simulink model "Day3_avoidance"  (R2022b)
settings: Solver=FixedStepAuto  StartTime=0.0  StopTime=inf  FixedStep=0.001  RelTol=1e-3  EnableMultiTasking=on
undefined symbols (not defined in the file): DiscIntNeverNeededParam
libraries: raspberrypiBasiclib x15, simulink x4, raspberrypisensorlib x1
settings Model: PacingRate=10  Creator=user  LastModifiedBy=user
settings SolverCC: PositivePriorityOrder=on
settings OptimizationCC: EnhancedBackFolding=on  PassReuseOutputArgsAs=Individual arguments  ZeroExternalMemoryAtStartup=off  ZeroInternalMemoryAtStartup=off  MaxStackSize=64  OptimizeBlockOrder=speed  DifferentSizesBufferReuse=on  OptimizationCustomize=off  EfficientTunableParamExpr=on
settings DebuggingCC: ParameterTunabilityLossMsg=error
settings HardwareCC: ProdBitPerPointer=32  ProdBitPerSizeT=32  ProdBitPerPtrDiffT=32  ProdLargestAtomicInteger=Long  ProdLargestAtomicFloat=Double  ProdWordSize=32  ProdLongLongMode=on  ProdHWDeviceType=ARM Compatible->ARM Cortex
settings RTWCC: Description=Embedded Coder  SystemTargetFile=ert.tlc  HardwareBoard=Raspberry Pi  TLCOptions="-aInlineSetEventsForThisBaseRateFcn=TLC_FALSE -aSuppressMultiTaskScheduler=TLC_FALSE  -aRateBasedStepFcn=0"  TemplateMakefile=ert_default_tmf  Toolchain=GNU GCC Embedded Linux  BuildConfiguration=Faster Runs
settings CodeAppCC: ForceParamTrailComments=on  IgnoreCustomStorageClasses=off  OperatorAnnotations=on  SimulinkDataObjDesc=on  SFDataObjDesc=on  InsertBlockDesc=on
settings ERTTargetCC: SupportVariableSizeSignals=on  ExtModeTransport=2  ExtModeStaticAlloc=on  ExtModeMexFile=ext_xcp  ExtModeIntrfLevel=Level2 - Open

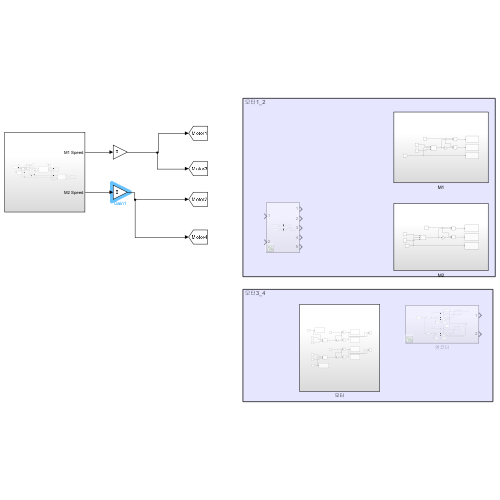
[thumbnail: Simulink's stored preview of the top-level diagram]
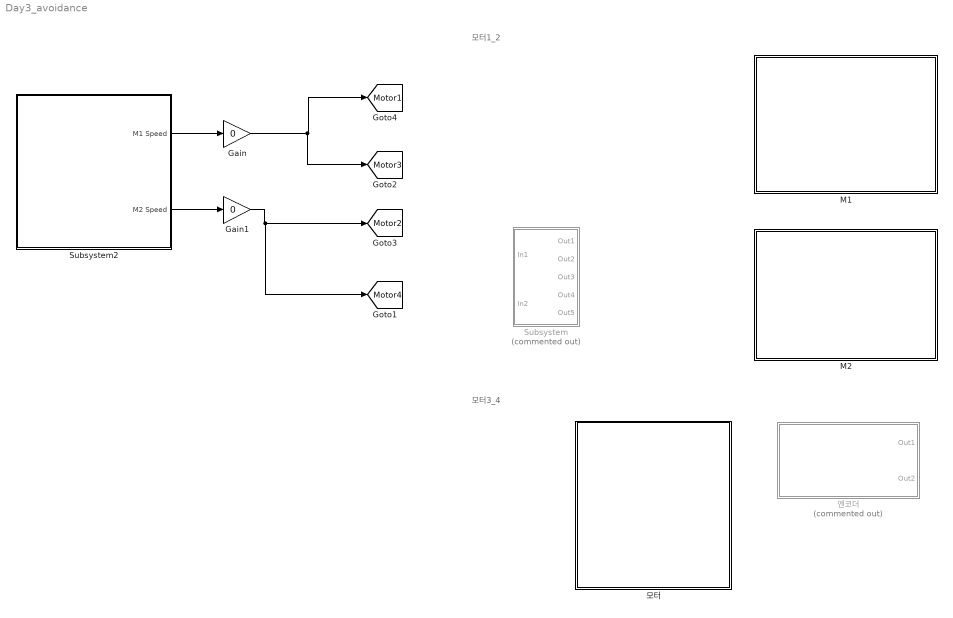
== system Day3_avoidance ==
  note: 모터1_2
  note: 모터3_4
  Gain : Gain  Gain=0
  Gain1 : Gain  Gain=0
  M1 : Subsystem
  M2 : Subsystem
  Subsystem : Subsystem  Commented=on
  Subsystem2 : Subsystem
  모터 : Subsystem
  엔코더 : Subsystem  Commented=on
  tag scope: Motor1=global, Motor2=global, Motor3=global, Motor4=global
  wires:
  Subsystem2/1(M1 Speed) -> Gain/1
  Subsystem2/2(M2 Speed) -> Gain1/1
  Gain/1 -> [Motor3], [Motor1]
  Gain1/1 -> [Motor4], [Motor2]

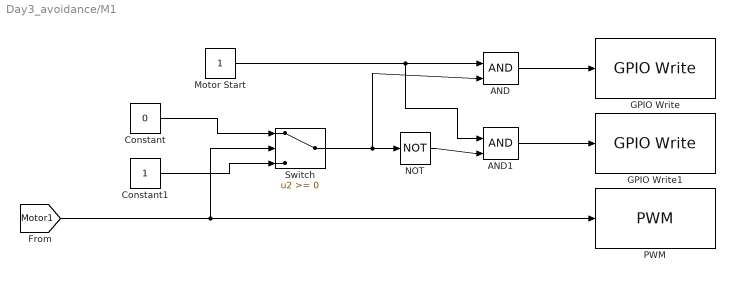
== system Day3_avoidance/M1 ==
  AND : Logic  IconShape=distinctive  AllPortsSameDT=off  OutDataTypeStr=boolean
  AND1 : Logic  IconShape=distinctive  AllPortsSameDT=off  OutDataTypeStr=boolean
  Constant : Constant  Value=0
  Constant1 : Constant
  GPIO Write : raspberrypiBasiclib/GPIO Write  board=Pi 4 Model B  gpio=15  direction=Output  blockPlatform=Raspberry Pi
  GPIO Write1 : raspberrypiBasiclib/GPIO Write  board=Pi 4 Model B  gpio=14  direction=Output  blockPlatform=Raspberry Pi
  Motor Start : Constant
  NOT : Logic  Operator=NOT  IconShape=distinctive  AllPortsSameDT=off  OutDataTypeStr=boolean
  PWM : raspberrypiBasiclib/PWM  board=Pi 4 Model B  Pin_=18  Frequency=50  blockPlatform=Raspberry Pi
  Switch : Switch  SaturateOnIntegerOverflow=off  InputSameDT=off
  wires:
  AND/1 -> GPIO Write/1
  Switch/1 -> AND/2, NOT/1
  Motor Start/1 -> AND1/1, AND/1
  AND1/1 -> GPIO Write1/1
  NOT/1 -> AND1/2
  [Motor1] -> Switch/2, PWM/1
  Constant/1 -> Switch/1
  Constant1/1 -> Switch/3

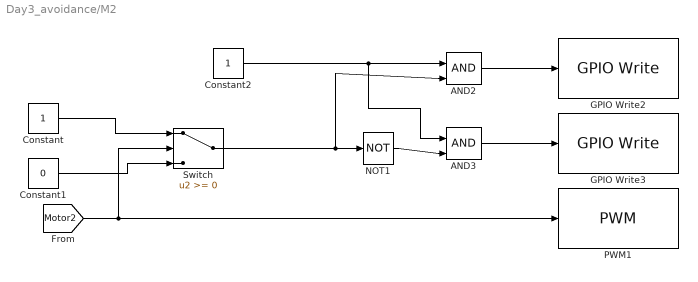
== system Day3_avoidance/M2 ==
  AND2 : Logic  IconShape=distinctive  AllPortsSameDT=off  OutDataTypeStr=boolean
  AND3 : Logic  IconShape=distinctive  AllPortsSameDT=off  OutDataTypeStr=boolean
  Constant : Constant
  Constant1 : Constant  Value=0
  Constant2 : Constant
  GPIO Write2 : raspberrypiBasiclib/GPIO Write  board=Pi 4 Model B  gpio=13  direction=Output  blockPlatform=Raspberry Pi
  GPIO Write3 : raspberrypiBasiclib/GPIO Write  board=Pi 4 Model B  gpio=6  direction=Output  blockPlatform=Raspberry Pi
  NOT1 : Logic  Operator=NOT  IconShape=distinctive  AllPortsSameDT=off  OutDataTypeStr=boolean
  PWM1 : raspberrypiBasiclib/PWM  board=Pi 4 Model B  Pin_=9  Frequency=50  blockPlatform=Raspberry Pi
  Switch : Switch  SaturateOnIntegerOverflow=off  InputSameDT=off
  wires:
  Constant2/1 -> AND3/1, AND2/1
  AND2/1 -> GPIO Write2/1
  AND3/1 -> GPIO Write3/1
  NOT1/1 -> AND3/2
  Switch/1 -> AND2/2, NOT1/1
  Constant1/1 -> Switch/3
  Constant/1 -> Switch/1
  [Motor2] -> Switch/2, PWM1/1

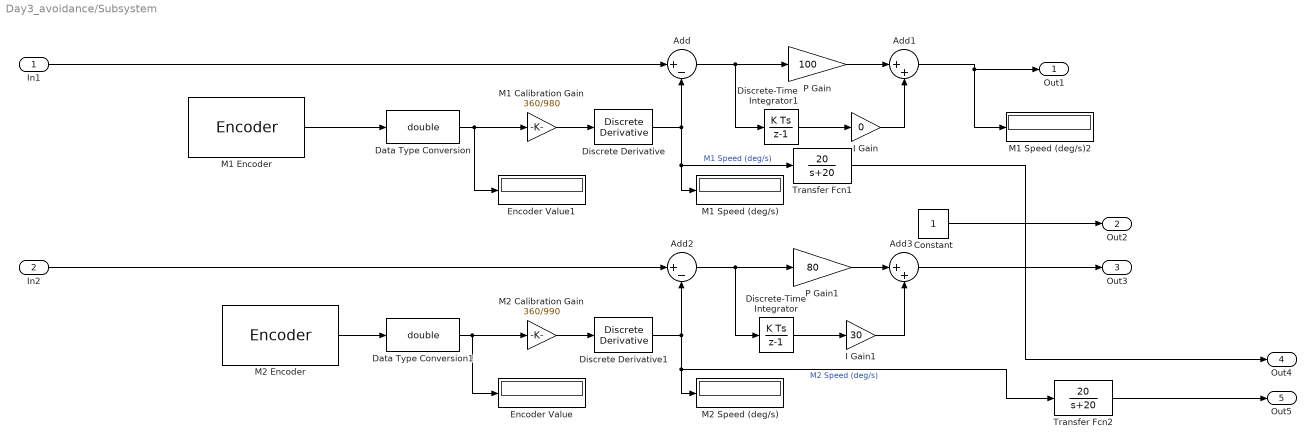
== system Day3_avoidance/Subsystem ==
  In1 : Inport
  In2 : Inport  Port=2
  Add : Sum  Inputs=|+-
  Add1 : Sum  Inputs=|++
  Add2 : Sum  Inputs=|+-
  Add3 : Sum  Inputs=|++
  Constant : Constant
  Data Type Conversion : DataTypeConversion  OutDataTypeStr=double  SaturateOnIntegerOverflow=off  RndMeth=Floor
  Data Type Conversion1 : DataTypeConversion  OutDataTypeStr=double  SaturateOnIntegerOverflow=off  RndMeth=Floor
  Discrete Derivative : simulink/Discrete/Discrete Derivative  gainval=1  ICPrevScaledInput=0.0  OutMin=[]  OutMax=[]  OutDataType=fixdt(1, 16)  OutScaling=2^-10  DoSatur=off
  Discrete Derivative1 : simulink/Discrete/Discrete Derivative  gainval=1.0  ICPrevScaledInput=0.0  OutMin=[]  OutMax=[]  OutDataType=fixdt(1, 16)  OutScaling=2^-10  DoSatur=off
  Discrete-Time Integrator : DiscreteIntegrator  SampleTime=-1  ICPrevOutput=DiscIntNeverNeededParam  ICPrevScaledInput=DiscIntNeverNeededParam
  Discrete-Time Integrator1 : DiscreteIntegrator  SampleTime=-1  ICPrevOutput=DiscIntNeverNeededParam  ICPrevScaledInput=DiscIntNeverNeededParam
  Encoder Value : Display
  Encoder Value1 : Display
  I Gain : Gain  Gain=0
  I Gain1 : Gain  Gain=30
  M1 Calibration Gain : Gain  Gain=360/980
  M1 Encoder : raspberrypiBasiclib/Encoder  BoardProperty=Pi 2 Model B  InputA=GPIO 10  InputB=GPIO 20  Mode=No reset  SampleTime=-1
  M1 Speed (deg/s) : Display
  M1 Speed (deg/s)2 : Display
  M2 Calibration Gain : Gain  Gain=360/990
  M2 Encoder : raspberrypiBasiclib/Encoder  BoardProperty=Pi 2 Model B  InputA=GPIO 17  InputB=GPIO 27  Mode=No reset  SampleTime=-1
  M2 Speed (deg/s) : Display
  P Gain : Gain  Gain=100
  P Gain1 : Gain  Gain=80
  Transfer Fcn1 : TransferFcn  Numerator=[20]  Denominator=[1 20]
  Transfer Fcn2 : TransferFcn  Numerator=[20]  Denominator=[1 20]
  Out1 : Outport
  Out2 : Outport  Port=2
  Out3 : Outport  Port=3
  Out4 : Outport  Port=4
  Out5 : Outport  Port=5
  wires:
  Discrete Derivative1/1 -> Add2/2, Transfer Fcn2/1, M2 Speed (deg/s)/1  "M2 Speed (deg/s)"
  M2 Calibration Gain/1 -> Discrete Derivative1/1
  Add1/1 -> Out1/1, M1 Speed (deg/s)2/1
  P Gain1/1 -> Add3/1
  Discrete-Time Integrator/1 -> I Gain1/1
  Add3/1 -> Out3/1
  M1 Encoder/1 -> Data Type Conversion/1
  Transfer Fcn1/1 -> Out4/1
  Transfer Fcn2/1 -> Out5/1
  In2/1 -> Add2/1
  Data Type Conversion/1 -> M1 Calibration Gain/1, Encoder Value1/1
  Constant/1 -> Out2/1
  Discrete Derivative/1 -> Add/2, Transfer Fcn1/1, M1 Speed (deg/s)/1  "M1 Speed (deg/s)"
  Discrete-Time Integrator1/1 -> I Gain/1
  Add/1 -> Discrete-Time Integrator1/1, P Gain/1
  M1 Calibration Gain/1 -> Discrete Derivative/1
  Add2/1 -> Discrete-Time Integrator/1, P Gain1/1
  I Gain1/1 -> Add3/2
  Data Type Conversion1/1 -> Encoder Value/1, M2 Calibration Gain/1
  I Gain/1 -> Add1/2
  M2 Encoder/1 -> Data Type Conversion1/1
  In1/1 -> Add/1
  P Gain/1 -> Add1/1

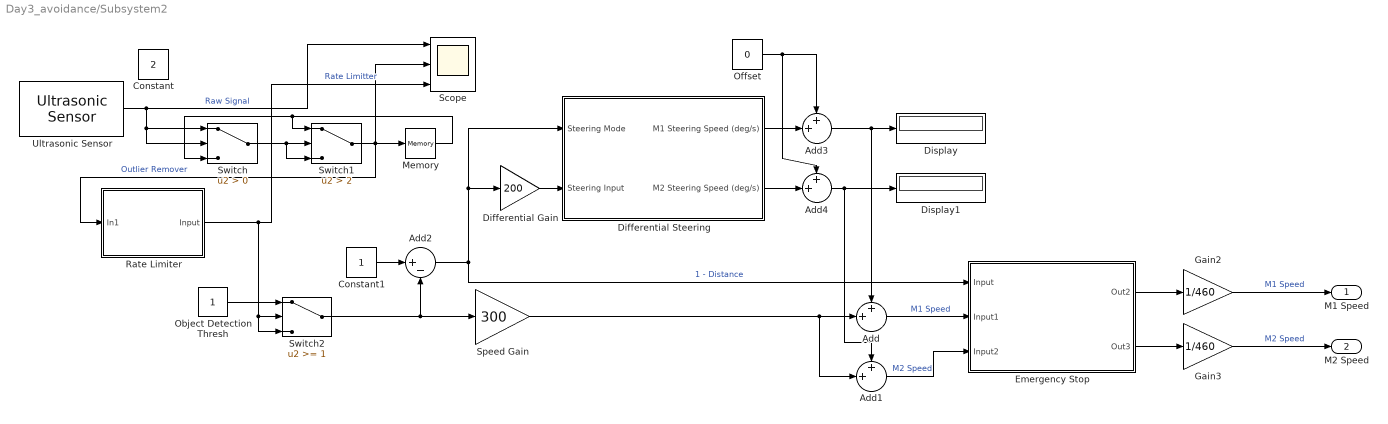
== system Day3_avoidance/Subsystem2 ==
  Add{,1,3..4} (4 alike) : Sum  Inputs=++|
  Add2 : Sum  Inputs=|+-
  Constant : Constant  Value=2
  Constant1 : Constant
  Differential Gain : Gain  Gain=200
  Differential Steering : Subsystem
  Display : Display
  Display1 : Display
  Emergency Stop : Subsystem
  Gain2 : Gain  Gain=1/460
  Gain3 : Gain  Gain=1/460
  Memory : Memory  InheritSampleTime=on  LinearizeMemory=on  LinearizeAsDelay=on
  Object Detection Thresh : Constant
  Offset : Constant  Value=0
  Rate Limiter : Subsystem
  Scope : Scope  NumInputPorts=3
  Speed Gain : Gain  Gain=300
  Switch : Switch  Criteria=u2 > Threshold  SaturateOnIntegerOverflow=off  InputSameDT=off
  Switch1 : Switch  Criteria=u2 > Threshold  Threshold=2  SaturateOnIntegerOverflow=off  InputSameDT=off
  Switch2 : Switch  Threshold=1  SaturateOnIntegerOverflow=off  InputSameDT=off
  Ultrasonic Sensor : raspberrypisensorlib/Ultrasonic Sensor  BoardProperty=Pi 4 Model B  NumSignalPins=2  TrigPin=GPIO 23  EchoPin=GPIO 24  SignalPin=GPIO 23  SampleTime=0.1  BlockPlatform=RASPBERRYPI
  M1 Speed : Outport
  M2 Speed : Outport  Port=2
  wires:
  Add3/1 -> Add/1, Display/1
  Add4/1 -> Display1/1, Add1/1
  Ultrasonic Sensor/1 -> Switch/2, Switch/1, Scope/1  "Raw Signal"
  Add2/1 -> Differential Gain/1, Differential Steering/1(Steering Mode), Emergency Stop/1(Input)  "1 - Distance"
  Differential Steering/2(M2 Steering Speed (deg/s)) -> Add4/2
  Switch/1 -> Switch1/3, Switch1/2
  Switch1/1 -> Memory/1, Scope/2, Rate Limiter/1(In1)  "Outlier Remover"
  Object Detection Thresh/1 -> Switch2/1
  Differential Steering/1(M1 Steering Speed (deg/s)) -> Add3/2
  Offset/1 -> Add4/1, Add3/1
  Gain2/1 -> M1 Speed/1  "M1 Speed"
  Constant1/1 -> Add2/1
  Differential Gain/1 -> Differential Steering/2(Steering Input)
  Gain3/1 -> M2 Speed/1  "M2 Speed"
  Switch2/1 -> Speed Gain/1, Add2/2
  Rate Limiter/1(Input) -> Scope/3, Switch2/3, Switch2/2  "Rate Limitter"
  Emergency Stop/1(Out2) -> Gain2/1
  Emergency Stop/2(Out3) -> Gain3/1
  Add/1 -> Emergency Stop/2(Input1)  "M1 Speed"
  Add1/1 -> Emergency Stop/3(Input2)  "M2 Speed"
  Memory/1 -> Switch/3, Switch1/1
  Speed Gain/1 -> Add1/2, Add/2

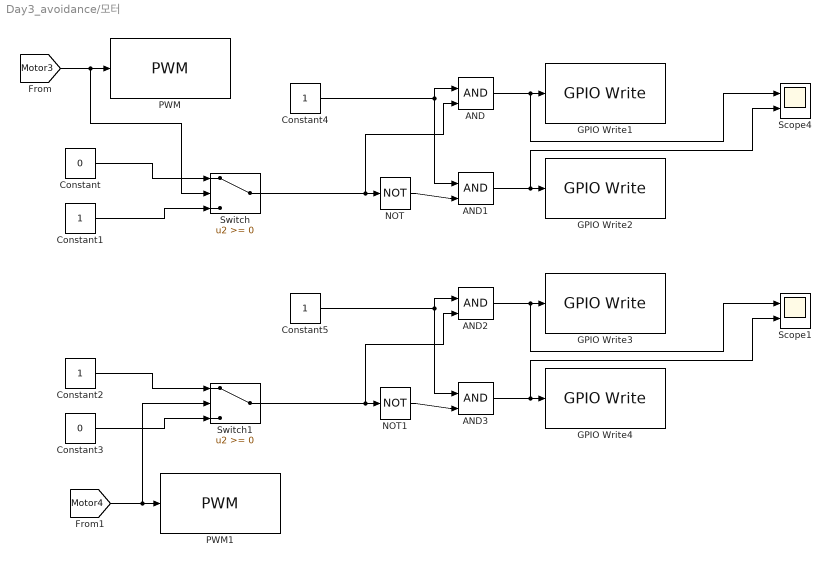
== system Day3_avoidance/모터 ==
  AND{,1..3} (4 alike) : Logic  IconShape=distinctive  AllPortsSameDT=off  OutDataTypeStr=boolean
  Constant : Constant  Value=0
  Constant{1..2,4..5} (4 alike) : Constant
  Constant3 : Constant  Value=0
  GPIO Write1 : raspberrypiBasiclib/GPIO Write  board=Pi 4 Model B  gpio=17  direction=Output  blockPlatform=Raspberry Pi
  GPIO Write2 : raspberrypiBasiclib/GPIO Write  board=Pi 4 Model B  gpio=27  direction=Output  blockPlatform=Raspberry Pi
  GPIO Write3 : raspberrypiBasiclib/GPIO Write  board=Pi 4 Model B  gpio=19  direction=Output  blockPlatform=Raspberry Pi
  GPIO Write4 : raspberrypiBasiclib/GPIO Write  board=Pi 4 Model B  gpio=26  direction=Output  blockPlatform=Raspberry Pi
  NOT : Logic  Operator=NOT  IconShape=distinctive  AllPortsSameDT=off  OutDataTypeStr=boolean
  NOT1 : Logic  Operator=NOT  IconShape=distinctive  AllPortsSameDT=off  OutDataTypeStr=boolean
  PWM : raspberrypiBasiclib/PWM  board=Pi 4 Model B  Pin_=25  Frequency=500  blockPlatform=Raspberry Pi
  PWM1 : raspberrypiBasiclib/PWM  board=Pi 4 Model B  Pin_=22  Frequency=500  blockPlatform=Raspberry Pi
  Scope1 : Scope  NumInputPorts=2
  Scope4 : Scope  NumInputPorts=2
  Switch : Switch  SaturateOnIntegerOverflow=off  InputSameDT=off
  Switch1 : Switch  SaturateOnIntegerOverflow=off  InputSameDT=off
  wires:
  Switch/1 -> AND/2, NOT/1
  Constant4/1 -> AND/1, AND1/1
  NOT/1 -> AND1/2
  AND/1 -> Scope4/1, GPIO Write1/1
  AND1/1 -> Scope4/2, GPIO Write2/1
  AND3/1 -> Scope1/2, GPIO Write4/1
  NOT1/1 -> AND3/2
  AND2/1 -> Scope1/1, GPIO Write3/1
  Constant5/1 -> AND2/1, AND3/1
  Switch1/1 -> AND2/2, NOT1/1
  [Motor3] -> Switch/2, PWM/1
  [Motor4] -> Switch1/2, PWM1/1
  Constant1/1 -> Switch/3
  Constant/1 -> Switch/1
  Constant2/1 -> Switch1/1
  Constant3/1 -> Switch1/3

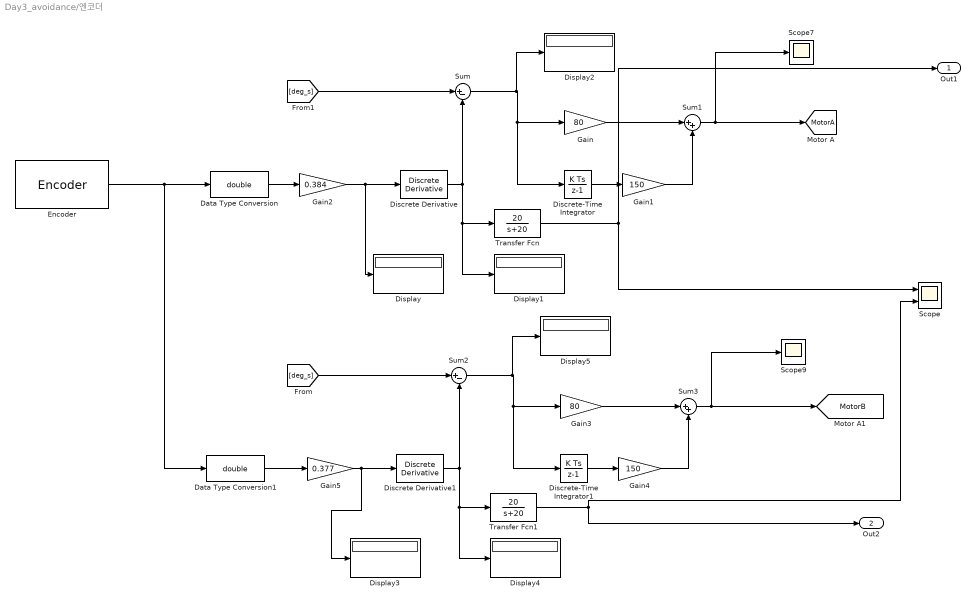
== system Day3_avoidance/엔코더 ==
  Data Type Conversion : DataTypeConversion  OutDataTypeStr=double  SaturateOnIntegerOverflow=off  RndMeth=Floor
  Data Type Conversion1 : DataTypeConversion  OutDataTypeStr=double  SaturateOnIntegerOverflow=off  RndMeth=Floor
  Discrete Derivative : simulink/Discrete/Discrete Derivative  gainval=1.0  ICPrevScaledInput=0.0  OutMin=[]  OutMax=[]  OutDataType=fixdt(1, 16)  OutScaling=2^-10  DoSatur=off
  Discrete Derivative1 : simulink/Discrete/Discrete Derivative  gainval=1.0  ICPrevScaledInput=0.0  OutMin=[]  OutMax=[]  OutDataType=fixdt(1, 16)  OutScaling=2^-10  DoSatur=off
  Discrete-Time Integrator : DiscreteIntegrator  SampleTime=-1  ICPrevOutput=DiscIntNeverNeededParam  ICPrevScaledInput=DiscIntNeverNeededParam
  Discrete-Time Integrator1 : DiscreteIntegrator  SampleTime=-1  ICPrevOutput=DiscIntNeverNeededParam  ICPrevScaledInput=DiscIntNeverNeededParam
  Display{,1..5} (6 alike) : Display
  Encoder : raspberrypiBasiclib/Encoder  BoardProperty=Pi 2 Model B  InputA=GPIO 11  InputB=GPIO 12  Mode=No reset  SampleTime=-1
  Gain : Gain  Gain=80
  Gain1 : Gain  Gain=150
  Gain2 : Gain  Gain=0.384
  Gain3 : Gain  Gain=80
  Gain4 : Gain  Gain=150
  Gain5 : Gain  Gain=0.377
  Scope : Scope  NumInputPorts=2
  Scope7 : Scope
  Scope9 : Scope
  Sum : Sum  Inputs=|+-
  Sum1 : Sum  Inputs=|++
  Sum2 : Sum  Inputs=|+-
  Sum3 : Sum  Inputs=|++
  Transfer Fcn : TransferFcn  Numerator=[20]  Denominator=[1 20]
  Transfer Fcn1 : TransferFcn  Numerator=[20]  Denominator=[1 20]
  Out1 : Outport
  Out2 : Outport  Port=2
  tag scope: MotorA=global, MotorB=global
  wires:
  Sum2/1 -> Display5/1, Discrete-Time Integrator1/1, Gain3/1
  Discrete Derivative/1 -> Transfer Fcn/1, Display1/1, Sum/2
  Discrete-Time Integrator/1 -> Gain1/1
  Gain1/1 -> Sum1/2
  Gain2/1 -> Discrete Derivative/1, Display/1
  Gain/1 -> Sum1/1
  Data Type Conversion/1 -> Gain2/1
  Sum/1 -> Display2/1, Discrete-Time Integrator/1, Gain/1
  Encoder/1 -> Data Type Conversion1/1, Data Type Conversion/1
  Sum1/1 -> [MotorA], Scope7/1
  [deg_s] -> Sum/1
  Sum3/1 -> [MotorB], Scope9/1
  Gain3/1 -> Sum3/1
  Gain4/1 -> Sum3/2
  Gain5/1 -> Discrete Derivative1/1, Display3/1
  Discrete Derivative1/1 -> Transfer Fcn1/1, Display4/1, Sum2/2
  [deg_s] -> Sum2/1
  Discrete-Time Integrator1/1 -> Gain4/1
  Data Type Conversion1/1 -> Gain5/1
  Transfer Fcn/1 -> Out1/1, Scope/1
  Transfer Fcn1/1 -> Out2/1, Scope/2

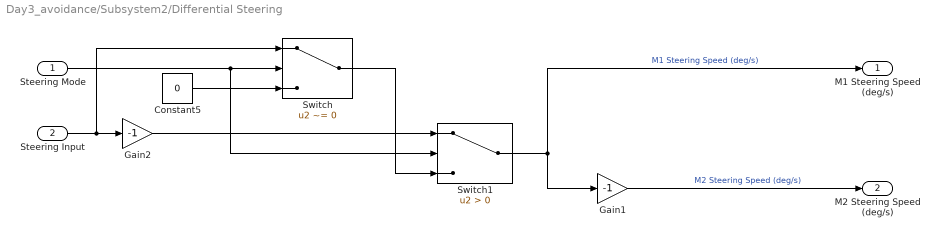
== system Day3_avoidance/Subsystem2/Differential Steering ==
  Steering Mode : Inport
  Steering Input : Inport  Port=2
  Constant5 : Constant  Value=0
  Gain1 : Gain  Gain=-1
  Gain2 : Gain  Gain=-1
  Switch : Switch  Criteria=u2 ~= 0  SaturateOnIntegerOverflow=off  InputSameDT=off
  Switch1 : Switch  Criteria=u2 > Threshold  SaturateOnIntegerOverflow=off  InputSameDT=off
  M1 Steering Speed (deg/s) : Outport
  M2 Steering Speed (deg/s) : Outport  Port=2
  wires:
  Gain1/1 -> M2 Steering Speed (deg/s)/1  "M2 Steering Speed (deg/s)"
  Switch1/1 -> M1 Steering Speed (deg/s)/1, Gain1/1  "M1 Steering Speed (deg/s)"
  Constant5/1 -> Switch/3
  Switch/1 -> Switch1/3
  Steering Mode/1 -> Switch1/2, Switch/2
  Steering Input/1 -> Switch/1, Gain2/1
  Gain2/1 -> Switch1/1

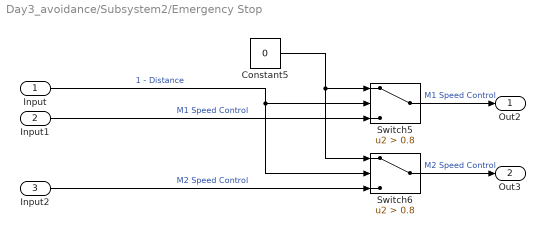
== system Day3_avoidance/Subsystem2/Emergency Stop ==
  Input : Inport
  Input1 : Inport  Port=2
  Input2 : Inport  Port=3
  Constant5 : Constant  Value=0
  Switch5 : Switch  Criteria=u2 > Threshold  Threshold=0.8  SaturateOnIntegerOverflow=off  InputSameDT=off
  Switch6 : Switch  Criteria=u2 > Threshold  Threshold=0.8  SaturateOnIntegerOverflow=off  InputSameDT=off
  Out2 : Outport
  Out3 : Outport  Port=2
  wires:
  Constant5/1 -> Switch6/1, Switch5/1
  Input/1 -> Switch6/2, Switch5/2  "1 - Distance"
  Switch6/1 -> Out3/1  "M2 Speed Control"
  Input2/1 -> Switch6/3  "M2 Speed Control"
  Switch5/1 -> Out2/1  "M1 Speed Control"
  Input1/1 -> Switch5/3  "M1 Speed Control"

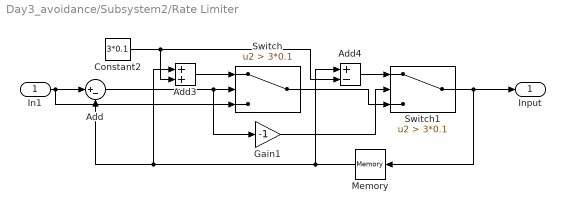
== system Day3_avoidance/Subsystem2/Rate Limiter ==
  In1 : Inport
  Add : Sum  Inputs=|+-
  Add3 : Sum
  Add4 : Sum  Inputs=+-
  Constant2 : Constant  Value=3*0.1
  Gain1 : Gain  Gain=-1
  Memory : Memory  InheritSampleTime=on  LinearizeMemory=on  LinearizeAsDelay=on
  Switch : Switch  Criteria=u2 > Threshold  Threshold=3*0.1  SaturateOnIntegerOverflow=off  InputSameDT=off
  Switch1 : Switch  Criteria=u2 > Threshold  Threshold=3*0.1  SaturateOnIntegerOverflow=off  InputSameDT=off
  Input : Outport
  wires:
  Switch/1 -> Switch1/3
  Constant2/1 -> Add4/2, Add3/2
  Switch1/1 -> Input/1, Memory/1
  Memory/1 -> Add/2, Add3/1, Add4/1
  Add4/1 -> Switch1/1
  Gain1/1 -> Switch1/2
  Add3/1 -> Switch/1
  Add/1 -> Switch/2, Gain1/1
  In1/1 -> Add/1, Switch/3
